simulink model "gm_sampleModel1936_2_sub"  (R2023a)
settings: Solver=VariableStepAuto  StartTime=0.0  StopTime=10.0  RelTol=1e-3
libraries: hdlsllib x1
settings Model: Creator=user1  LastModifiedBy=user1
settings OptimizationCC: BlockReduction=off  ConditionallyExecuteInputs=off
settings DebuggingCC: InheritedTsInSrcMsg=none

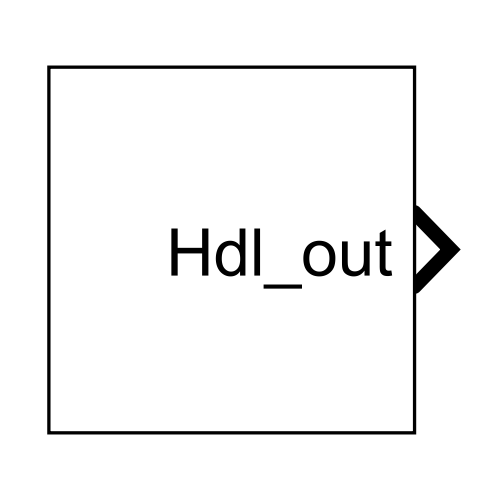
[thumbnail: Simulink's stored preview of the top-level diagram]
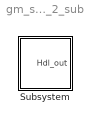
== system gm_sampleModel1936_2_sub ==
  Subsystem : Subsystem

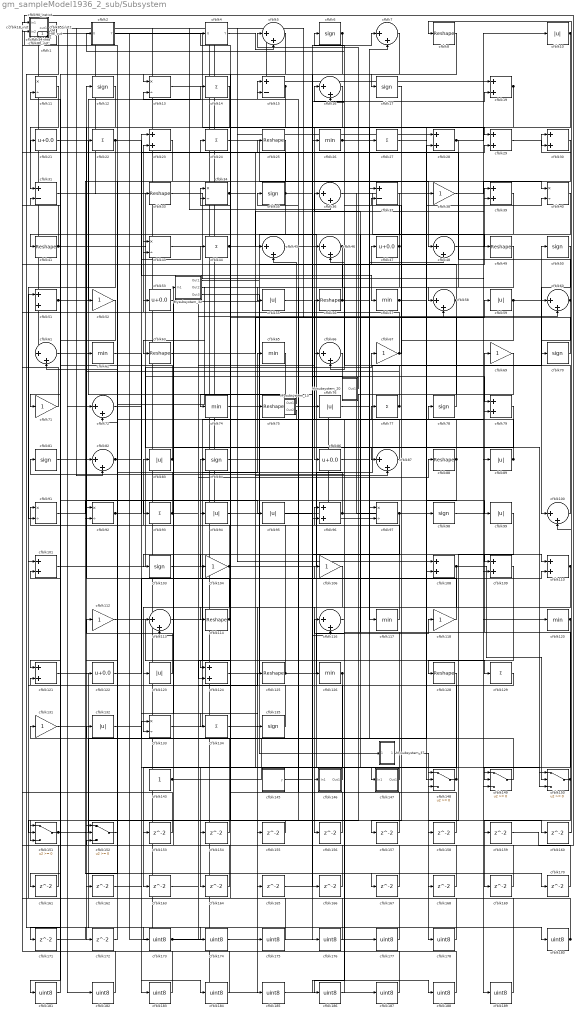
== system gm_sampleModel1936_2_sub/Subsystem ==
  Mysubsystem_13 : Subsystem
  Mysubsystem_20 : Subsystem
  Mysubsystem_32 : Subsystem
  Mysubsystem_37 : Subsystem
  cfblk1 : hdlsllib/Logic and Bit Operations/Interval Test  IntervalClosedRight=on  uplimit=0.5  IntervalClosedLeft=on  lowlimit=-0.5  OutDataTypeStr=uint8
  cfblk{10,55,59,76,83,89,94..95,99,123,132} (11 alike) : Abs  OutDataTypeStr=uint8  SaturateOnIntegerOverflow=off
  cfblk{5,7,16,36,45..46,48,58,60..61,66,72,82,87,100,113,116} (17 alike) : Sum  Inputs=|++  OutDataTypeStr=uint8
  cfblk{19,23,28..30,39,51,79,96,101,108..110,121,124} (15 alike) : Sum  OutDataTypeStr=uint8
  cfblk102_inst : Subsystem
  cfblk{6,12,17,35,50,70,78,81,84,98,103,135} (12 alike) : Signum
  cfblk{38,52,67,69,71,104,106,112,118,131} (10 alike) : Gain  OutDataTypeStr=uint8
  cfblk107_inst : Subsystem
  cfblk{11,13,34,40,43,91..92,97,133} (9 alike) : Product  Inputs=*/  OutDataTypeStr=uint8  RndMeth=Zero  SaturateOnIntegerOverflow=on
  cfblk111_inst : Subsystem
  cfblk{8,25,33,41,49,56,63,75,88,114,125,128} (12 alike) : Reshape
  cfblk115_inst : Subsystem
  cfblk{26,57,62,65,74,117,120,126} (8 alike) : MinMax  OutDataTypeStr=uint8
  cfblk{21,47,53,86,122} (5 alike) : Bias  Bias=0.0  SaturateOnIntegerOverflow=off
  cfblk{14,22,24,27,44,77,93,129,134} (9 alike) : Sum  Inputs=+  OutDataTypeStr=uint8
  cfblk130_inst : Subsystem
  cfblk136_inst : Subsystem
  cfblk143 : Constant  OutDataTypeStr=uint8  SampleTime=-1
  cfblk145 : Subsystem  mask(Counter Free-Running){NumBits=double(16), tsamp=double(-1)}
      mask prompts: NumBits "Simulink:masks:NumberOfBits_MP"; tsamp "Simulink:masks:SampleTime_MP"
      mask help: Simulink:masks:CounterFreeRunning_MD
  cfblk146 : Subsystem
  cfblk147 : Subsystem
  cfblk{148..152} (5 alike) : Switch  OutDataTypeStr=uint8  SaturateOnIntegerOverflow=off  InputSameDT=off
  cfblk15 : Sum  Inputs=+-  OutDataTypeStr=uint8
  cfblk{153..172} (20 alike) : Delay  SampleTime=1
  cfblk{173..178,180..189} (16 alike) : DataTypeConversion  OutDataTypeStr=uint8  SaturateOnIntegerOverflow=off  RndMeth=Floor
  cfblk18_inst : Subsystem
  cfblk2 : Subsystem  mask(Detect Fall Nonpositive){vinit=double(0), InputProcessing=Elements as channels (sample based), OutDataTypeStr=uint8}
      mask prompts: vinit "Simulink:masks:InitialCondition_MP"; InputProcessing "Simulink:masks:InputProcessing_MP"; OutDataTypeStr "Simulink:masks:OutputDataType_MP"
      mask help: Simulink:masks:DetectFallNonpositive_MD
      mask init:
      | InputProcessing = 'Elements as channels (sample based)';
      | OutDataTypeStr = 'uint8';
      | vinit = double(0);
      mask TypeOptions InputProcessing: Simulink:masks:ColumnsAsChannelsFrameBased | Simulink:masks:ElementsAsChannelsSampleBased
      mask TypeOptions OutDataTypeStr: Simulink:masks:uint8 | Simulink:masks:boolean
      mask Display: fprintf('U <= 0\n&  NOT\nU/z <= 0')
  cfblk31 : Sum  Inputs=+-  OutDataTypeStr=uint8
  cfblk37 : Sum  Inputs=+-  OutDataTypeStr=uint8
  cfblk4 : Subsystem  mask(Detect Fall Nonpositive){vinit=double(0), InputProcessing=Elements as channels (sample based), OutDataTypeStr=uint8}
      mask prompts: vinit "Simulink:masks:InitialCondition_MP"; InputProcessing "Simulink:masks:InputProcessing_MP"; OutDataTypeStr "Simulink:masks:OutputDataType_MP"
      mask help: Simulink:masks:DetectFallNonpositive_MD
      mask init:
      | InputProcessing = 'Elements as channels (sample based)';
      | OutDataTypeStr = 'uint8';
      | vinit = double(0);
      mask TypeOptions InputProcessing: Simulink:masks:ColumnsAsChannelsFrameBased | Simulink:masks:ElementsAsChannelsSampleBased
      mask TypeOptions OutDataTypeStr: Simulink:masks:uint8 | Simulink:masks:boolean
      mask Display: fprintf('U <= 0\n&  NOT\nU/z <= 0')
  cfblk54_inst : Subsystem
  cfblk80_inst : Subsystem
  cfblk85_inst : Subsystem
  cfblk90_inst : Subsystem
  Hdl_out : Outport  OutDataTypeStr=uint8  SampleTime=1
  wires:
  Mysubsystem_13/1(Out1) -> cfblk45/2
  Mysubsystem_13/2(Out2) -> Mysubsystem_32/1(In1)
  Mysubsystem_20/1(Out1) -> cfblk5/1
  Mysubsystem_32/1(Out1) -> cfblk149/2
  Mysubsystem_32/2(Out2) -> cfblk151/3
  Mysubsystem_32/3(Out3) -> Mysubsystem_37/1(In1)
  Mysubsystem_37/1(Out1) -> cfblk178/1
  cfblk1/1 -> cfblk173/1
  cfblk10/1 -> cfblk86/1, cfblk74/1
  cfblk100/1 -> cfblk46/2
  cfblk101/1 -> cfblk67/1
  cfblk102_inst/1(out1) -> cfblk187/1
  cfblk103/1 -> cfblk129/1
  cfblk104/1 -> cfblk83/1, cfblk50/1, cfblk148/3, cfblk133/2
  cfblk106/1 -> cfblk185/1
  cfblk107_inst/1(out1) -> cfblk182/1
  cfblk108/1 -> cfblk150/2, cfblk123/1
  cfblk109/1 -> cfblk158/1
  cfblk11/1 -> cfblk31/1
  cfblk110/1 -> cfblk8/1, cfblk156/1
  cfblk111_inst/1(out1) -> cfblk60/2, cfblk45/1
  cfblk112/1 -> cfblk166/1
  cfblk113/1 -> cfblk69/1
  cfblk114/1 -> cfblk84/1, cfblk12/1
  cfblk115_inst/1(out1) -> cfblk108/1
  cfblk116/1 -> cfblk56/1
  cfblk117/1 -> cfblk11/2
  cfblk118/1 -> cfblk35/1
  cfblk12/1 -> cfblk172/1
  cfblk120/1 -> cfblk30/1, cfblk149/3
  cfblk121/1 -> cfblk160/1
  cfblk122/1 -> cfblk110/2
  cfblk123/1 -> cfblk112/1
  cfblk124/1 -> cfblk39/1
  cfblk125/1 -> cfblk118/1, cfblk24/1
  cfblk126/1 -> cfblk164/1, cfblk163/1
  cfblk128/1 -> cfblk186/1
  cfblk129/1 -> cfblk121/2
  cfblk13/1 -> cfblk97/1
  cfblk130_inst/1(out1) -> cfblk72/1, cfblk51/2, cfblk36/2
  cfblk131/1 -> cfblk180/1
  cfblk132/1 -> cfblk170/1
  cfblk133/1 -> cfblk65/1
  cfblk134/1 -> cfblk165/1
  cfblk135/1 -> cfblk82/1
  cfblk136_inst/1(out1) -> cfblk19/1
  cfblk14/1 -> cfblk41/1
  cfblk143/1 -> cfblk28/2, cfblk26/1
  cfblk145/1(y) -> cfblk176/1
  cfblk146/1(Out1) -> cfblk91/1
  cfblk147/1(Out1) -> cfblk136_inst/2(in2)
  cfblk148/1 -> cfblk76/1, cfblk51/1
  cfblk149/1 -> cfblk132/1
  cfblk15/1 -> cfblk181/1, cfblk13/2
  cfblk150/1 -> cfblk81/1, cfblk79/2, cfblk36/1, cfblk169/1
  cfblk151/1 -> cfblk133/1, cfblk27/1
  cfblk152/1 -> cfblk92/1
  cfblk153/1 -> cfblk90_inst/2(in2)
  cfblk154/1 -> cfblk101/2
  cfblk155/1 -> cfblk152/1
  cfblk156/1 -> cfblk46/1
  cfblk157/1 -> cfblk34/1
  cfblk158/1 -> cfblk15/1
  cfblk159/1 -> cfblk136_inst/1(in1)
  cfblk16/1 -> cfblk93/1
  cfblk160/1 -> cfblk100/2
  cfblk161/1 -> cfblk85_inst/1(in1)
  cfblk162/1 -> cfblk184/1
  cfblk163/1 -> cfblk66/1
  cfblk164/1 -> cfblk130_inst/2(in2)
  cfblk165/1 -> cfblk19/2
  cfblk166/1 -> cfblk18_inst/2(in2)
  cfblk167/1 -> cfblk152/3
  cfblk168/1 -> cfblk116/1
  cfblk169/1 -> cfblk23/2
  cfblk17/1 -> cfblk157/1
  cfblk170/1 -> cfblk96/1
  cfblk171/1 -> cfblk174/1
  cfblk172/1 -> cfblk72/2
  cfblk173/1 -> cfblk58/2, cfblk47/1, cfblk125/1
  cfblk174/1 -> cfblk1/1
  cfblk175/1 -> cfblk94/1
  cfblk176/1 -> cfblk54_inst/1(in1)
  cfblk177/1 -> cfblk54_inst/2(in2)
  cfblk178/1 -> cfblk80_inst/2(in2)
  cfblk18_inst/1(out1) -> cfblk61/1
  cfblk180/1 -> cfblk115_inst/1(in1), cfblk101/1
  cfblk181/1 -> cfblk131/1
  cfblk182/1 -> cfblk80_inst/1(in1)
  cfblk183/1 -> cfblk107_inst/1(in1)
  cfblk184/1 -> cfblk107_inst/2(in2)
  cfblk185/1 -> cfblk188/1
  cfblk186/1 -> cfblk106/1
  cfblk187/1 -> cfblk21/1
  cfblk188/1 -> cfblk102_inst/1(in1)
  cfblk189/1 -> cfblk102_inst/2(in2)
  cfblk19/1 -> cfblk151/1, cfblk114/1, cfblk108/2
  cfblk2/1(Y) -> cfblk189/1
  cfblk21/1 -> cfblk110/1
  cfblk22/1 -> cfblk91/2, cfblk57/1
  cfblk23/1 -> cfblk152/2
  cfblk24/1 -> cfblk48/1
  cfblk25/1 -> cfblk162/1
  cfblk26/1 -> cfblk48/2, cfblk29/1
  cfblk27/1 -> cfblk99/1
  cfblk28/1 -> cfblk58/1, cfblk10/1
  cfblk29/1 -> cfblk30/2
  cfblk30/1 -> cfblk104/1
  cfblk31/1 -> cfblk79/1
  cfblk33/1 -> cfblk89/1
  cfblk34/1 -> cfblk87/2, cfblk29/2, cfblk154/1
  cfblk35/1 -> cfblk148/1, cfblk111_inst/2(in2), cfblk92/2
  cfblk36/1 -> cfblk49/1
  cfblk37/1 -> cfblk146/1(In1)
  cfblk38/1 -> cfblk40/1
  cfblk39/1 -> cfblk122/1
  cfblk4/1(Y) -> cfblk5/2
  cfblk40/1 -> cfblk71/1
  cfblk41/1 -> cfblk18_inst/1(in1), cfblk150/1
  cfblk43/1 -> cfblk117/1
  cfblk44/1 -> cfblk39/2, cfblk147/1(In1)
  cfblk45/1 -> cfblk7/1
  cfblk46/1 -> cfblk16/1, cfblk155/1
  cfblk47/1 -> cfblk66/2, cfblk63/1, cfblk2/1(U)
  cfblk48/1 -> cfblk120/1
  cfblk49/1 -> cfblk55/1
  cfblk5/1 -> cfblk121/1
  cfblk50/1 -> cfblk100/1
  cfblk51/1 -> cfblk159/1, cfblk14/1
  cfblk52/1 -> cfblk161/1
  cfblk53/1 -> cfblk135/1
  cfblk54_inst/1(out1) -> cfblk175/1
  cfblk55/1 -> cfblk168/1
  cfblk56/1 -> cfblk90_inst/1(in1), cfblk7/2, cfblk16/2
  cfblk57/1 -> cfblk148/2, cfblk40/2
  cfblk58/1 -> cfblk151/2, cfblk43/1
  cfblk59/1 -> cfblk87/1, cfblk60/1
  cfblk6/1 -> cfblk13/1, cfblk126/1
  cfblk60/1 -> cfblk70/1, cfblk22/1
  cfblk61/1 -> cfblk183/1
  cfblk62/1 -> cfblk134/1
  cfblk63/1 -> cfblk59/1
  cfblk65/1 -> cfblk124/1
  cfblk66/1 -> cfblk96/2
  cfblk67/1 -> cfblk37/2, cfblk130_inst/1(in1)
  cfblk69/1 -> cfblk153/1
  cfblk7/1 -> cfblk124/2
  cfblk70/1 -> cfblk4/1(U)
  cfblk71/1 -> cfblk85_inst/2(in2)
  cfblk72/1 -> cfblk23/1
  cfblk74/1 -> cfblk77/1
  cfblk75/1 -> cfblk98/1, cfblk97/2, cfblk38/1
  cfblk76/1 -> cfblk109/1
  cfblk77/1 -> cfblk43/2, cfblk62/1
  cfblk78/1 -> cfblk6/1
  cfblk79/1 -> cfblk113/2
  cfblk8/1 -> cfblk17/1
  cfblk80_inst/1(out1) -> cfblk33/1
  cfblk81/1 -> cfblk167/1
  cfblk82/1 -> cfblk25/1, cfblk52/1
  cfblk83/1 -> cfblk31/2, cfblk113/1
  cfblk84/1 -> cfblk116/2
  cfblk85_inst/1(out1) -> cfblk82/2, cfblk28/1
  cfblk86/1 -> cfblk78/1
  cfblk87/1 -> cfblk37/1
  cfblk88/1 -> cfblk53/1, cfblk171/1
  cfblk89/1 -> cfblk75/1, cfblk115_inst/2(in2)
  cfblk90_inst/1(out1) -> cfblk177/1, cfblk11/1
  cfblk91/1 -> cfblk95/1
  cfblk92/1 -> cfblk150/3, cfblk44/1
  cfblk93/1 -> cfblk88/1, cfblk111_inst/1(in1)
  cfblk94/1 -> cfblk34/2
  cfblk95/1 -> cfblk149/1
  cfblk96/1 -> cfblk61/2, cfblk15/2
  cfblk97/1 -> cfblk103/1, Hdl_out/1
  cfblk98/1 -> cfblk109/2
  cfblk99/1 -> cfblk128/1

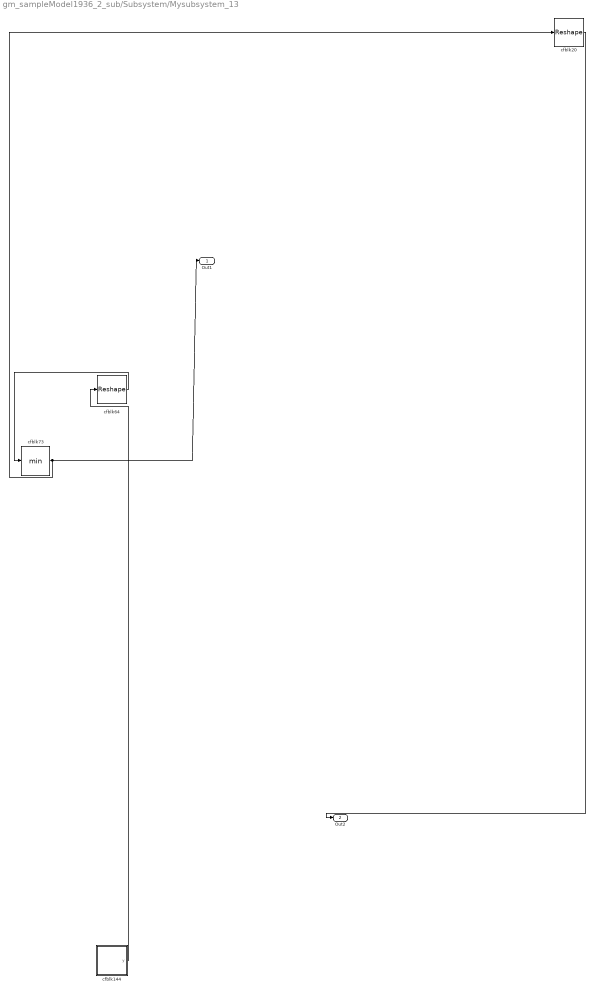
== system gm_sampleModel1936_2_sub/Subsystem/Mysubsystem_13 ==
  cfblk144 : Subsystem  mask(Counter Limited){uplimit=double(7), tsamp=double(-1)}
      mask prompts: uplimit "Simulink:masks:UpperLimit_MP"; tsamp "Simulink:masks:SampleTime_MP"
      mask help: Simulink:masks:CounterLimited_MD
      mask init:
      | nbits = double(8);
      | tsamp = double(-1);
      | uplimit = double(7);
  cfblk20 : Reshape
  cfblk64 : Reshape
  cfblk73 : MinMax
  Out1 : Outport  SampleTime=1
  Out2 : Outport  Port=2  SampleTime=1
  wires:
  cfblk144/1(y) -> cfblk64/1
  cfblk20/1 -> Out2/1
  cfblk64/1 -> cfblk73/1
  cfblk73/1 -> cfblk20/1, Out1/1

== system gm_sampleModel1936_2_sub/Subsystem/Mysubsystem_20 ==
  cfblk142 : Subsystem  mask(Counter Limited){uplimit=double(7), tsamp=double(-1)}
      mask prompts: uplimit "Simulink:masks:UpperLimit_MP"; tsamp "Simulink:masks:SampleTime_MP"
      mask help: Simulink:masks:CounterLimited_MD
      mask init:
      | nbits = double(8);
      | tsamp = double(-1);
      | uplimit = double(7);
  cfblk68 : Gain
  cfblk9 : Abs  SaturateOnIntegerOverflow=off
  Out1 : Outport  SampleTime=1
  wires:
  cfblk142/1(y) -> cfblk9/1
  cfblk68/1 -> Out1/1
  cfblk9/1 -> cfblk68/1

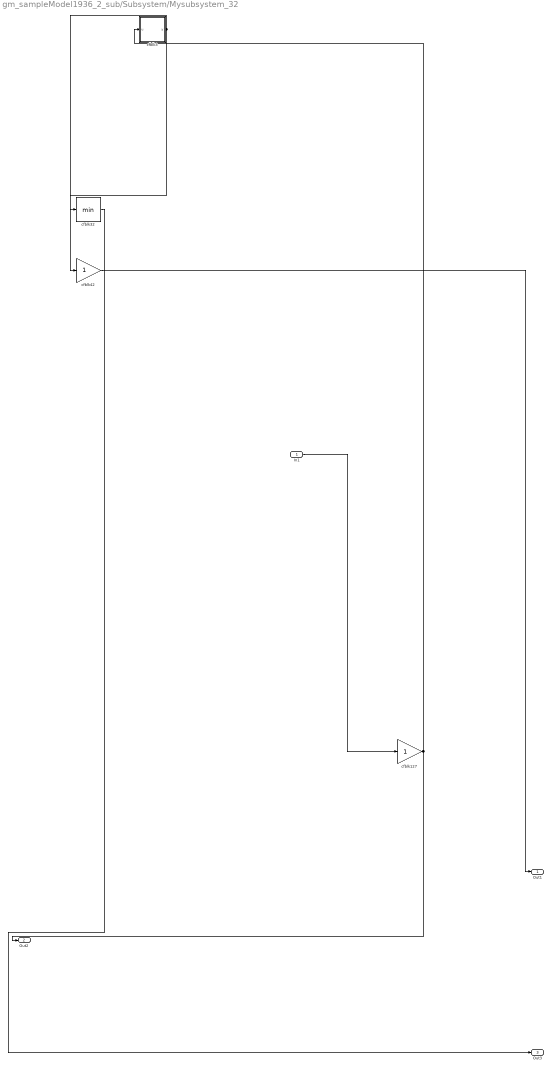
== system gm_sampleModel1936_2_sub/Subsystem/Mysubsystem_32 ==
  In1 : Inport  OutDataTypeStr=uint8  PortDimensions=1  SampleTime=1
  cfblk127 : Gain
  cfblk3 : Subsystem  mask(Compare To Zero){relop=<=, OutDataTypeStr=boolean, ZeroCross=on}
      mask prompts: relop "Simulink:masks:Operator_MP"; OutDataTypeStr "Simulink:masks:OutputDataType_MP"; ZeroCross "Simulink:masks:EnableZerocrossingDetection_MP"
      mask help: Simulink:masks:CompareToZero_MD
      mask init:
      | OutDataTypeStr = 'boolean';
      | ZeroCross = 'on';
      | blkName = 'sampleModel1936_2_sub/Subsystem/Mysubsystem_32/cfblk3';
      | relop = '<=';
      | setValue = 'boolean';
      mask TypeOptions relop: == | ~= | < | <= | >= | >
      mask TypeOptions OutDataTypeStr: Simulink:masks:uint8 | Simulink:masks:boolean
      mask Callback ZeroCross: sl('zeroCrossEnable', gcbh);
      mask Display: disp([relop,' 0'])
  cfblk32 : MinMax
  cfblk42 : Gain
  Out1 : Outport  SampleTime=1
  Out2 : Outport  Port=2  SampleTime=1
  Out3 : Outport  Port=3  SampleTime=1
  wires:
  In1/1 -> cfblk127/1
  cfblk127/1 -> cfblk3/1(u), Out2/1
  cfblk3/1(y) -> cfblk42/1, cfblk32/1
  cfblk32/1 -> Out3/1
  cfblk42/1 -> Out1/1

== system gm_sampleModel1936_2_sub/Subsystem/Mysubsystem_37 ==
  In1 : Inport  OutDataTypeStr=boolean  PortDimensions=1  SampleTime=1
  cfblk105 : Abs  SaturateOnIntegerOverflow=off
  cfblk179 : DataTypeConversion  OutDataTypeStr=uint8  SaturateOnIntegerOverflow=off  RndMeth=Floor
  Out1 : Outport  SampleTime=1
  wires:
  In1/1 -> cfblk179/1
  cfblk105/1 -> Out1/1
  cfblk179/1 -> cfblk105/1

== system gm_sampleModel1936_2_sub/Subsystem/cfblk102_inst ==
  in1 : Inport  OutDataTypeStr=uint8  SampleTime=1
  in2 : Inport  Port=2  OutDataTypeStr=uint8  SampleTime=1
  mul_cfblk102_dotp_mulcomp : Product  Inputs=**  OutDataTypeStr=uint8  SampleTime=1
  out1 : Outport  OutDataTypeStr=uint8  SampleTime=1
  wires:
  in1/1 -> mul_cfblk102_dotp_mulcomp/1
  in2/1 -> mul_cfblk102_dotp_mulcomp/2
  mul_cfblk102_dotp_mulcomp/1 -> out1/1

== system gm_sampleModel1936_2_sub/Subsystem/cfblk107_inst ==
  in1 : Inport  OutDataTypeStr=uint8  SampleTime=1
  in2 : Inport  Port=2  OutDataTypeStr=uint8  SampleTime=1
  mul_cfblk107_dotp_mulcomp : Product  Inputs=**  OutDataTypeStr=uint8  SampleTime=1
  out1 : Outport  OutDataTypeStr=uint8  SampleTime=1
  wires:
  in1/1 -> mul_cfblk107_dotp_mulcomp/1
  in2/1 -> mul_cfblk107_dotp_mulcomp/2
  mul_cfblk107_dotp_mulcomp/1 -> out1/1

== system gm_sampleModel1936_2_sub/Subsystem/cfblk111_inst ==
  in1 : Inport  OutDataTypeStr=uint8  SampleTime=1
  in2 : Inport  Port=2  OutDataTypeStr=uint8  SampleTime=1
  mul_cfblk111_dotp_mulcomp : Product  Inputs=**  OutDataTypeStr=uint8  SampleTime=1
  out1 : Outport  OutDataTypeStr=uint8  SampleTime=1
  wires:
  in1/1 -> mul_cfblk111_dotp_mulcomp/1
  in2/1 -> mul_cfblk111_dotp_mulcomp/2
  mul_cfblk111_dotp_mulcomp/1 -> out1/1

== system gm_sampleModel1936_2_sub/Subsystem/cfblk115_inst ==
  in1 : Inport  OutDataTypeStr=uint8  SampleTime=1
  in2 : Inport  Port=2  OutDataTypeStr=uint8  SampleTime=1
  mul_cfblk115_dotp_mulcomp : Product  Inputs=**  OutDataTypeStr=uint8  SampleTime=1
  out1 : Outport  OutDataTypeStr=uint8  SampleTime=1
  wires:
  in1/1 -> mul_cfblk115_dotp_mulcomp/1
  in2/1 -> mul_cfblk115_dotp_mulcomp/2
  mul_cfblk115_dotp_mulcomp/1 -> out1/1

== system gm_sampleModel1936_2_sub/Subsystem/cfblk130_inst ==
  in1 : Inport  OutDataTypeStr=uint8  SampleTime=1
  in2 : Inport  Port=2  OutDataTypeStr=uint8  SampleTime=1
  mul_cfblk130_dotp_mulcomp : Product  Inputs=**  OutDataTypeStr=uint8  SampleTime=1
  out1 : Outport  OutDataTypeStr=uint8  SampleTime=1
  wires:
  in1/1 -> mul_cfblk130_dotp_mulcomp/1
  in2/1 -> mul_cfblk130_dotp_mulcomp/2
  mul_cfblk130_dotp_mulcomp/1 -> out1/1

== system gm_sampleModel1936_2_sub/Subsystem/cfblk136_inst ==
  in1 : Inport  OutDataTypeStr=uint8  SampleTime=1
  in2 : Inport  Port=2  OutDataTypeStr=uint8  SampleTime=1
  mul_cfblk136_dotp_mulcomp : Product  Inputs=**  OutDataTypeStr=uint8  SampleTime=1
  out1 : Outport  OutDataTypeStr=uint8  SampleTime=1
  wires:
  in1/1 -> mul_cfblk136_dotp_mulcomp/1
  in2/1 -> mul_cfblk136_dotp_mulcomp/2
  mul_cfblk136_dotp_mulcomp/1 -> out1/1

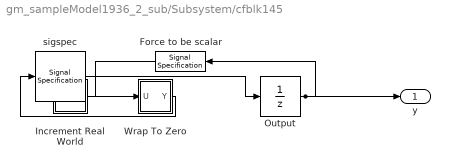
== system gm_sampleModel1936_2_sub/Subsystem/cfblk145 ==
  Force to be scalar : SignalSpecification  DisableCoverage=on  Dimensions=1
  Increment Real World : Subsystem  mask(Real World Value Increment){}
      mask help: Simulink:masks:RealWorldValueIncrement_MD
      mask Display: disp('V++')
  Output : UnitDelay  InitialCondition=0.0  SampleTime=tsamp  HasFrameUpgradeWarning=on
  Wrap To Zero : Subsystem  mask(Wrap To Zero){Threshold=double(65535)}
      mask prompts: Threshold "Simulink:masks:Threshold_MP"
      mask help: Simulink:masks:WrapToZero_MD
  sigspec : SignalSpecification  OutDataTypeStr=uint16  Dimensions=1
  y : Outport  SampleTime=1
  wires:
  Force to be scalar/1 -> Increment Real World/1(u)
  Increment Real World/1(y) -> Wrap To Zero/1(U)
  Output/1 -> Force to be scalar/1, y/1
  Wrap To Zero/1(Y) -> sigspec/1
  sigspec/1 -> Output/1

== system gm_sampleModel1936_2_sub/Subsystem/cfblk146 ==
  In1 : Inport  OutDataTypeStr=uint8  PortDimensions=1  SampleTime=1
  Out1 : Outport  SampleTime=1
  wires:
  In1/1 -> Out1/1

== system gm_sampleModel1936_2_sub/Subsystem/cfblk147 ==
  In1 : Inport  OutDataTypeStr=uint8  PortDimensions=1  SampleTime=1
  Out1 : Outport  SampleTime=1
  wires:
  In1/1 -> Out1/1

== system gm_sampleModel1936_2_sub/Subsystem/cfblk18_inst ==
  in1 : Inport  OutDataTypeStr=uint8  SampleTime=1
  in2 : Inport  Port=2  OutDataTypeStr=uint8  SampleTime=1
  mul_cfblk18_dotp_mulcomp : Product  Inputs=**  OutDataTypeStr=uint8  SampleTime=1
  out1 : Outport  OutDataTypeStr=uint8  SampleTime=1
  wires:
  in1/1 -> mul_cfblk18_dotp_mulcomp/1
  in2/1 -> mul_cfblk18_dotp_mulcomp/2
  mul_cfblk18_dotp_mulcomp/1 -> out1/1

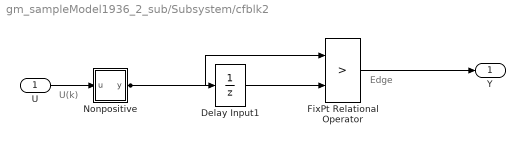
== system gm_sampleModel1936_2_sub/Subsystem/cfblk2 ==
  note: U(k)
  note: Edge
  U : Inport  OutDataTypeStr=uint8  SampleTime=1
  Delay Input1 : UnitDelay  Description=Store in Global RAM  DisableCoverage=on  InitialCondition=vinit  SampleTime=-1  HasFrameUpgradeWarning=on
  FixPt Relational Operator : RelationalOperator  Operator=>  OutDataTypeStr=fixdt(0, 8)  ZeroCross=off  InputSameDT=off
  Nonpositive : Subsystem  mask(Compare To Zero){relop=<=, OutDataTypeStr=boolean, ZeroCross=off}
      mask prompts: relop "Simulink:masks:Operator_MP"; OutDataTypeStr "Simulink:masks:OutputDataType_MP"; ZeroCross "Simulink:masks:EnableZerocrossingDetection_MP"
      mask help: Simulink:masks:CompareToZero_MD
      mask init:
      | OutDataTypeStr = 'boolean';
      | ZeroCross = 'off';
      | blkName = 'sampleModel1936_2_sub/Subsystem/cfblk2/Nonpositive';
      | relop = '<=';
      | setValue = 'boolean';
      mask TypeOptions relop: == | ~= | < | <= | >= | >
      mask TypeOptions OutDataTypeStr: Simulink:masks:uint8 | Simulink:masks:boolean
      mask Callback ZeroCross: sl('zeroCrossEnable', gcbh);
      mask Display: disp([relop,' 0'])
  Y : Outport  SampleTime=1
  wires:
  U/1 -> Nonpositive/1(u)
  Delay Input1/1 -> FixPt Relational Operator/2
  FixPt Relational Operator/1 -> Y/1
  Nonpositive/1(y) -> FixPt Relational Operator/1, Delay Input1/1

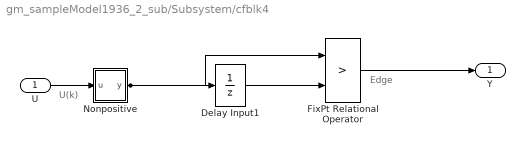
== system gm_sampleModel1936_2_sub/Subsystem/cfblk4 ==
  note: U(k)
  note: Edge
  U : Inport  OutDataTypeStr=uint8  SampleTime=1
  Delay Input1 : UnitDelay  Description=Store in Global RAM  DisableCoverage=on  InitialCondition=vinit  SampleTime=-1  HasFrameUpgradeWarning=on
  FixPt Relational Operator : RelationalOperator  Operator=>  OutDataTypeStr=fixdt(0, 8)  ZeroCross=off  InputSameDT=off
  Nonpositive : Subsystem  mask(Compare To Zero){relop=<=, OutDataTypeStr=boolean, ZeroCross=off}
      mask prompts: relop "Simulink:masks:Operator_MP"; OutDataTypeStr "Simulink:masks:OutputDataType_MP"; ZeroCross "Simulink:masks:EnableZerocrossingDetection_MP"
      mask help: Simulink:masks:CompareToZero_MD
      mask init:
      | OutDataTypeStr = 'boolean';
      | ZeroCross = 'off';
      | blkName = 'sampleModel1936_2_sub/Subsystem/cfblk4/Nonpositive';
      | relop = '<=';
      | setValue = 'boolean';
      mask TypeOptions relop: == | ~= | < | <= | >= | >
      mask TypeOptions OutDataTypeStr: Simulink:masks:uint8 | Simulink:masks:boolean
      mask Callback ZeroCross: sl('zeroCrossEnable', gcbh);
      mask Display: disp([relop,' 0'])
  Y : Outport  SampleTime=1
  wires:
  U/1 -> Nonpositive/1(u)
  Delay Input1/1 -> FixPt Relational Operator/2
  FixPt Relational Operator/1 -> Y/1
  Nonpositive/1(y) -> FixPt Relational Operator/1, Delay Input1/1

== system gm_sampleModel1936_2_sub/Subsystem/cfblk54_inst ==
  in1 : Inport  OutDataTypeStr=uint8  SampleTime=1
  in2 : Inport  Port=2  OutDataTypeStr=uint8  SampleTime=1
  mul_cfblk54_dotp_mulcomp : Product  Inputs=**  OutDataTypeStr=uint8  SampleTime=1
  out1 : Outport  OutDataTypeStr=uint8  SampleTime=1
  wires:
  in1/1 -> mul_cfblk54_dotp_mulcomp/1
  in2/1 -> mul_cfblk54_dotp_mulcomp/2
  mul_cfblk54_dotp_mulcomp/1 -> out1/1

== system gm_sampleModel1936_2_sub/Subsystem/cfblk80_inst ==
  in1 : Inport  OutDataTypeStr=uint8  SampleTime=1
  in2 : Inport  Port=2  OutDataTypeStr=uint8  SampleTime=1
  mul_cfblk80_dotp_mulcomp : Product  Inputs=**  OutDataTypeStr=uint8  SampleTime=1
  out1 : Outport  OutDataTypeStr=uint8  SampleTime=1
  wires:
  in1/1 -> mul_cfblk80_dotp_mulcomp/1
  in2/1 -> mul_cfblk80_dotp_mulcomp/2
  mul_cfblk80_dotp_mulcomp/1 -> out1/1

== system gm_sampleModel1936_2_sub/Subsystem/cfblk85_inst ==
  in1 : Inport  OutDataTypeStr=uint8  SampleTime=1
  in2 : Inport  Port=2  OutDataTypeStr=uint8  SampleTime=1
  mul_cfblk85_dotp_mulcomp : Product  Inputs=**  OutDataTypeStr=uint8  SampleTime=1
  out1 : Outport  OutDataTypeStr=uint8  SampleTime=1
  wires:
  in1/1 -> mul_cfblk85_dotp_mulcomp/1
  in2/1 -> mul_cfblk85_dotp_mulcomp/2
  mul_cfblk85_dotp_mulcomp/1 -> out1/1

== system gm_sampleModel1936_2_sub/Subsystem/cfblk90_inst ==
  in1 : Inport  OutDataTypeStr=uint8  SampleTime=1
  in2 : Inport  Port=2  OutDataTypeStr=uint8  SampleTime=1
  mul_cfblk90_dotp_mulcomp : Product  Inputs=**  OutDataTypeStr=uint8  SampleTime=1
  out1 : Outport  OutDataTypeStr=uint8  SampleTime=1
  wires:
  in1/1 -> mul_cfblk90_dotp_mulcomp/1
  in2/1 -> mul_cfblk90_dotp_mulcomp/2
  mul_cfblk90_dotp_mulcomp/1 -> out1/1

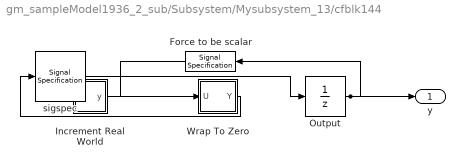
== system gm_sampleModel1936_2_sub/Subsystem/Mysubsystem_13/cfblk144 ==
  Force to be scalar : SignalSpecification  DisableCoverage=on  Dimensions=1
  Increment Real World : Subsystem  mask(Real World Value Increment){}
      mask help: Simulink:masks:RealWorldValueIncrement_MD
      mask Display: disp('V++')
  Output : UnitDelay  InitialCondition=0.0  SampleTime=tsamp  HasFrameUpgradeWarning=on
  Wrap To Zero : Subsystem  mask(Wrap To Zero){Threshold=double(7)}
      mask prompts: Threshold "Simulink:masks:Threshold_MP"
      mask help: Simulink:masks:WrapToZero_MD
  sigspec : SignalSpecification  OutDataTypeStr=uint8  Dimensions=1
  y : Outport  SampleTime=1
  wires:
  Force to be scalar/1 -> Increment Real World/1(u)
  Increment Real World/1(y) -> Wrap To Zero/1(U)
  Output/1 -> Force to be scalar/1, y/1
  Wrap To Zero/1(Y) -> sigspec/1
  sigspec/1 -> Output/1

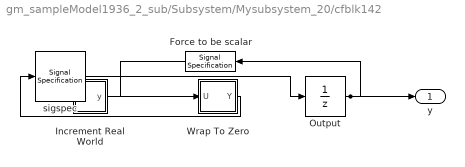
== system gm_sampleModel1936_2_sub/Subsystem/Mysubsystem_20/cfblk142 ==
  Force to be scalar : SignalSpecification  DisableCoverage=on  Dimensions=1
  Increment Real World : Subsystem  mask(Real World Value Increment){}
      mask help: Simulink:masks:RealWorldValueIncrement_MD
      mask Display: disp('V++')
  Output : UnitDelay  InitialCondition=0.0  SampleTime=tsamp  HasFrameUpgradeWarning=on
  Wrap To Zero : Subsystem  mask(Wrap To Zero){Threshold=double(7)}
      mask prompts: Threshold "Simulink:masks:Threshold_MP"
      mask help: Simulink:masks:WrapToZero_MD
  sigspec : SignalSpecification  OutDataTypeStr=uint8  Dimensions=1
  y : Outport  SampleTime=1
  wires:
  Force to be scalar/1 -> Increment Real World/1(u)
  Increment Real World/1(y) -> Wrap To Zero/1(U)
  Output/1 -> Force to be scalar/1, y/1
  Wrap To Zero/1(Y) -> sigspec/1
  sigspec/1 -> Output/1

== system gm_sampleModel1936_2_sub/Subsystem/Mysubsystem_32/cfblk3 ==
  u : Inport  OutDataTypeStr=fixdt(0, 16, 7)  SampleTime=1
  Compare : RelationalOperator  Operator=<=  OutDataTypeStr=boolean
  Constant : Constant  DisableCoverage=on  Value=0  OutDataTypeStr=Inherit: Inherit via back propagation  SampleTime=-1  PreserveConstantTs=on
  y : Outport  SampleTime=1
  wires:
  u/1 -> Compare/1
  Compare/1 -> y/1
  Constant/1 -> Compare/2

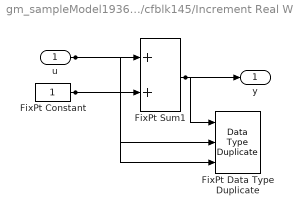
== system gm_sampleModel1936_2_sub/Subsystem/cfblk145/Increment Real World ==
  u : Inport  OutDataTypeStr=uint16  SampleTime=1
  FixPt Constant : Constant  DisableCoverage=on  OutDataTypeStr=Inherit: Inherit via back propagation  SampleTime=-1
  FixPt Data Type Duplicate : DataTypeDuplicate  DisableCoverage=on  NumInputPorts=3
  FixPt Sum1 : Sum  InputSameDT=on  OutDataTypeStr=Inherit: Inherit via back propagation  LockScale=on
  y : Outport  SampleTime=1
  wires:
  u/1 -> FixPt Sum1/1, FixPt Data Type Duplicate/2
  FixPt Constant/1 -> FixPt Sum1/2, FixPt Data Type Duplicate/3
  FixPt Sum1/1 -> FixPt Data Type Duplicate/1, y/1

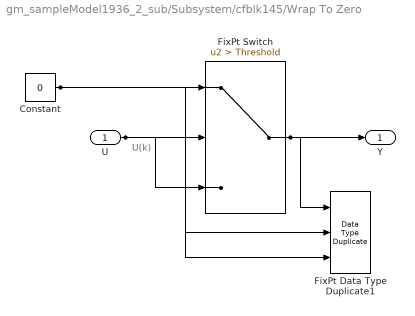
== system gm_sampleModel1936_2_sub/Subsystem/cfblk145/Wrap To Zero ==
  note: U(k)
  U : Inport  OutDataTypeStr=uint16  SampleTime=1
  Constant : Constant  DisableCoverage=on  Value=0  OutDataTypeStr=Inherit: Inherit via back propagation  SampleTime=-1
  FixPt Data Type Duplicate1 : DataTypeDuplicate  DisableCoverage=on  NumInputPorts=3
  FixPt Switch : Switch  Criteria=u2 > Threshold  Threshold=Threshold  OutDataTypeStr=Inherit: Inherit via back propagation  ZeroCross=off  SaturateOnIntegerOverflow=off  InputSameDT=off
  Y : Outport  SampleTime=1
  wires:
  U/1 -> FixPt Switch/3, FixPt Switch/2, FixPt Data Type Duplicate1/2
  Constant/1 -> FixPt Switch/1, FixPt Data Type Duplicate1/3
  FixPt Switch/1 -> FixPt Data Type Duplicate1/1, Y/1

== system gm_sampleModel1936_2_sub/Subsystem/cfblk2/Nonpositive ==
  u : Inport  OutDataTypeStr=uint8  SampleTime=1
  Compare : RelationalOperator  Operator=<=  OutDataTypeStr=boolean  ZeroCross=off
  Constant : Constant  DisableCoverage=on  Value=0  OutDataTypeStr=Inherit: Inherit via back propagation  SampleTime=-1  PreserveConstantTs=on
  y : Outport  SampleTime=1
  wires:
  u/1 -> Compare/1
  Compare/1 -> y/1
  Constant/1 -> Compare/2

== system gm_sampleModel1936_2_sub/Subsystem/cfblk4/Nonpositive ==
  u : Inport  OutDataTypeStr=uint8  SampleTime=1
  Compare : RelationalOperator  Operator=<=  OutDataTypeStr=boolean  ZeroCross=off
  Constant : Constant  DisableCoverage=on  Value=0  OutDataTypeStr=Inherit: Inherit via back propagation  SampleTime=-1  PreserveConstantTs=on
  y : Outport  SampleTime=1
  wires:
  u/1 -> Compare/1
  Compare/1 -> y/1
  Constant/1 -> Compare/2

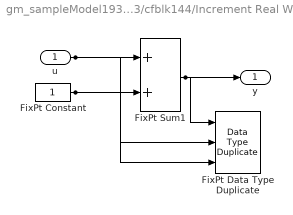
== system gm_sampleModel1936_2_sub/Subsystem/Mysubsystem_13/cfblk144/Increment Real World ==
  u : Inport  OutDataTypeStr=uint8  SampleTime=1
  FixPt Constant : Constant  DisableCoverage=on  OutDataTypeStr=Inherit: Inherit via back propagation  SampleTime=-1
  FixPt Data Type Duplicate : DataTypeDuplicate  DisableCoverage=on  NumInputPorts=3
  FixPt Sum1 : Sum  InputSameDT=on  OutDataTypeStr=Inherit: Inherit via back propagation  LockScale=on
  y : Outport  SampleTime=1
  wires:
  u/1 -> FixPt Sum1/1, FixPt Data Type Duplicate/2
  FixPt Constant/1 -> FixPt Sum1/2, FixPt Data Type Duplicate/3
  FixPt Sum1/1 -> FixPt Data Type Duplicate/1, y/1

== system gm_sampleModel1936_2_sub/Subsystem/Mysubsystem_13/cfblk144/Wrap To Zero ==
  note: U(k)
  U : Inport  OutDataTypeStr=uint8  SampleTime=1
  Constant : Constant  DisableCoverage=on  Value=0  OutDataTypeStr=Inherit: Inherit via back propagation  SampleTime=-1
  FixPt Data Type Duplicate1 : DataTypeDuplicate  DisableCoverage=on  NumInputPorts=3
  FixPt Switch : Switch  Criteria=u2 > Threshold  Threshold=Threshold  OutDataTypeStr=Inherit: Inherit via back propagation  ZeroCross=off  SaturateOnIntegerOverflow=off  InputSameDT=off
  Y : Outport  SampleTime=1
  wires:
  U/1 -> FixPt Switch/3, FixPt Switch/2, FixPt Data Type Duplicate1/2
  Constant/1 -> FixPt Switch/1, FixPt Data Type Duplicate1/3
  FixPt Switch/1 -> FixPt Data Type Duplicate1/1, Y/1

== system gm_sampleModel1936_2_sub/Subsystem/Mysubsystem_20/cfblk142/Increment Real World ==
  u : Inport  OutDataTypeStr=uint8  SampleTime=1
  FixPt Constant : Constant  DisableCoverage=on  OutDataTypeStr=Inherit: Inherit via back propagation  SampleTime=-1
  FixPt Data Type Duplicate : DataTypeDuplicate  DisableCoverage=on  NumInputPorts=3
  FixPt Sum1 : Sum  InputSameDT=on  OutDataTypeStr=Inherit: Inherit via back propagation  LockScale=on
  y : Outport  SampleTime=1
  wires:
  u/1 -> FixPt Sum1/1, FixPt Data Type Duplicate/2
  FixPt Constant/1 -> FixPt Sum1/2, FixPt Data Type Duplicate/3
  FixPt Sum1/1 -> FixPt Data Type Duplicate/1, y/1

== system gm_sampleModel1936_2_sub/Subsystem/Mysubsystem_20/cfblk142/Wrap To Zero ==
  note: U(k)
  U : Inport  OutDataTypeStr=uint8  SampleTime=1
  Constant : Constant  DisableCoverage=on  Value=0  OutDataTypeStr=Inherit: Inherit via back propagation  SampleTime=-1
  FixPt Data Type Duplicate1 : DataTypeDuplicate  DisableCoverage=on  NumInputPorts=3
  FixPt Switch : Switch  Criteria=u2 > Threshold  Threshold=Threshold  OutDataTypeStr=Inherit: Inherit via back propagation  ZeroCross=off  SaturateOnIntegerOverflow=off  InputSameDT=off
  Y : Outport  SampleTime=1
  wires:
  U/1 -> FixPt Switch/3, FixPt Switch/2, FixPt Data Type Duplicate1/2
  Constant/1 -> FixPt Switch/1, FixPt Data Type Duplicate1/3
  FixPt Switch/1 -> FixPt Data Type Duplicate1/1, Y/1
